simulink model "simu_ejemplo"  (R2021a)
settings: Solver=VariableStepAuto  StartTime=0.0  StopTime=5  RelTol=1e-3
values from neighbouring files (symbols this model uses):
  A = [1 1 ; -4 -3]    [Bessel_ejemplo.m]    (also in ITAE_ejemplo.m; ejemplo.m = [ 0 1 0; 0 0 1; -1 -5 -6])
  B = [0;2]    [Bessel_ejemplo.m]    (also in ITAE_ejemplo.m; ejemplo.m = [0;0;1])
  K = acker(A,B,[s1 s2])    [Bessel_ejemplo.m]    (also in ITAE_ejemplo.m; ejemplo.m = [alfa3-a3 alfa2-a2 alfa1-a1])
settings Model: Creator=pierr  LastModifiedBy=pierr

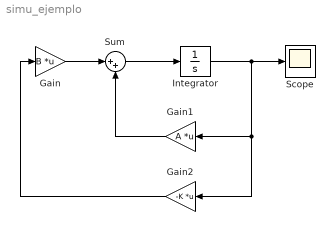
== system simu_ejemplo ==
  Gain : Gain  Gain=B  Multiplication=Matrix(K*u)
  Gain1 : Gain  Gain=A  Multiplication=Matrix(K*u)
  Gain2 : Gain  Gain=-K  Multiplication=Matrix(K*u)
  Integrator : Integrator  InitialCondition=[0;0.1]
  Scope : Scope
  Sum : Sum  Inputs=|++
  wires:
  Sum/1 -> Integrator/1
  Gain/1 -> Sum/1
  Gain1/1 -> Sum/2
  Gain2/1 -> Gain/1
  Integrator/1 -> Scope/1, Gain1/1, Gain2/1
